simulink model "Turbofan_Model"  (R2025b)
settings: Solver=VariableStepAuto  StartTime=0.0  StopTime=1  RelTol=1e-3
libraries: aerolibpropulsion2 x1
settings Model: Creator=afone  LastModifiedBy=afone

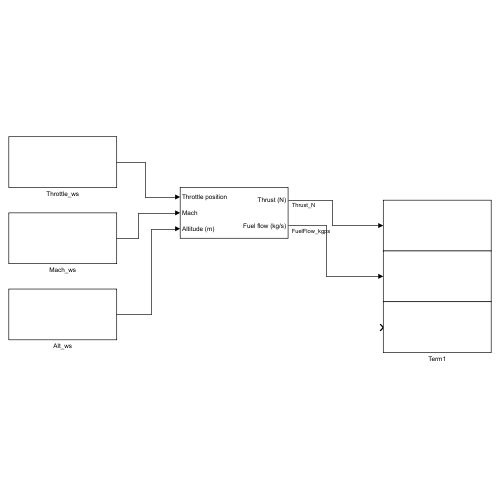
[thumbnail: Simulink's stored preview of the top-level diagram]
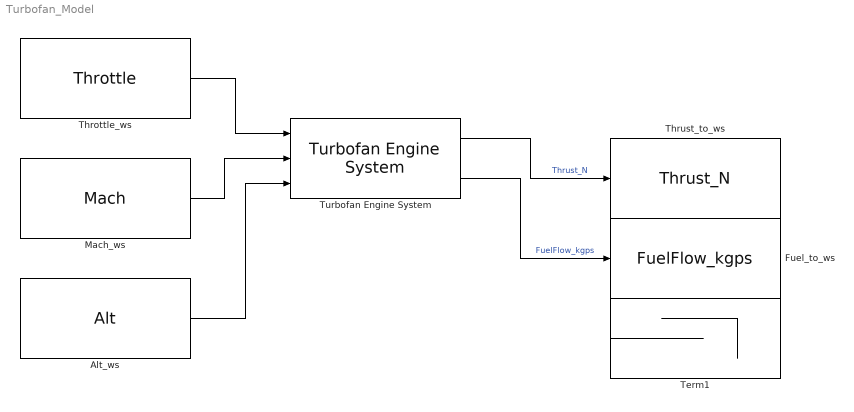
== system Turbofan_Model ==
  Alt_ws : FromWorkspace  VariableName=Alt
  Fuel_to_ws : ToWorkspace  VariableName=FuelFlow_kgps  SaveFormat=Timeseries  SampleTime=-1
  Mach_ws : FromWorkspace  VariableName=Mach
  Term1 : Terminator
  Throttle_ws : FromWorkspace  VariableName=Throttle
  Thrust_to_ws : ToWorkspace  VariableName=Thrust_N  SaveFormat=Timeseries  SampleTime=-1
  Turbofan Engine System : aerolibpropulsion2/Turbofan Engine System  units=Metric (MKS)  ic_source=Internal  IC=0  Fmax=120000  tau=1e-07  SFC=1e-05  Nt=0.9
  wires:
  Throttle_ws/1 -> Turbofan Engine System/1
  Mach_ws/1 -> Turbofan Engine System/2
  Alt_ws/1 -> Turbofan Engine System/3
  Turbofan Engine System/1 -> Thrust_to_ws/1  "Thrust_N"
  Turbofan Engine System/2 -> Fuel_to_ws/1  "FuelFlow_kgps"
